simulink library "ExperimentLibrary"  (R2014b)
settings: Solver=ode45  StartTime=0.0  StopTime=10.0  RelTol=1e-3
libraries: simulink x16, ExperimentLibrary x10, simulink_extras x2
settings Model: CovModelRefEnable=off  CovSFcnEnable=on  Creator=oortg  LastModifiedBy=OortG

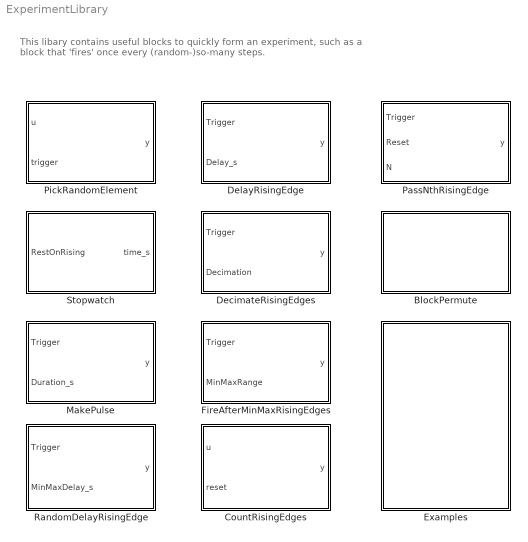
== system ExperimentLibrary ==
  note: This libary contains useful blocks to quickly form an experiment, such as a block that 'fires' once every (random-)so-many steps.
  BlockPermute : Subsystem
  CountRisingEdges : MATLAB Function  TreatAsAtomicUnit=on
      settings: PermitHierarchicalResolution=ParametersOnly
  DecimateRisingEdges : Subsystem
  DelayRisingEdge : Subsystem
  Examples : Subsystem
  FireAfterMinMaxRisingEdges : Subsystem
  MakePulse : Subsystem
  PassNthRisingEdge : Subsystem
  PickRandomElement : MATLAB Function  TreatAsAtomicUnit=on
      settings: PermitHierarchicalResolution=ParametersOnly
  RandomDelayRisingEdge : Subsystem
  Stopwatch : Subsystem

== system ExperimentLibrary/BlockPermute ==
  note: Given vectors in1, in2, in3 and in4, this block will, sequentially, output
      | all combinations of various elements of the inputs in a random order,
      | such that, after N=len(in1)*len(in2)*len(in3)*len(in4)*Ntimes, each combination was
      | output exactly Ntimes times. It is allowed to keep any inX unconnected;
      | this makes the block work for only the remaining inputs.
      |
      | Ntimes should low enough that the total number of combinations offered, N, is
      | less or equal to 1000. If not, Ntimes is reduced until the condition is
      | satisfied. Ntimes can be changed at any time; if so, a new experiment
      | with fresh a random order is started.
      |
      | Each time a rising edge on trigger is encountered, a new combination is
      | generated. Each time a rising edge on trigger_back is generated, the
      | previous combination is output (a simultaneous rising edge on both will
      | continue offering the current combination). For the first time sample of
      | the model (i.e., directly after pressing 'run'), the value of
      | trigger/trigger_back are considered; if nonzero this is seen as a rising
      | edge (this allows for generating the first combination at sample 1
      | already, thus skipping the 'initial value').
      |
      | When N combination are output (i.e., we're finished), a new round is
      | started with a freshly randomized order. The number of completed
      | rounds is returned as 3rd argument in the 'info' output.
      |
      | The first combination is only shown as soon as the first trigger appeared.
      | Because the block needs to output always, there is an initialValue input,
      | which is used as the output values before the first trigger (and also
      | after a enough trigger_back events). It defaults to zero if left empty.
      |
      | It is allowed to change the input values inX during the experiment (though,
      | not the length of the vectors). Internally, only the indices of all combinations
      | are permuted, not the input values themselves. So the block keeps
      | working, keeping in mind which elements of the input arrays had been used
      | or not).
      |
      | On a rising edge of reset, the internal state of the block is reset. It
      | is NOT a level reset though (contrary to most other blocks in the
      | ExperimentLibrary), so even when the reset input is non-zero, the block
      | functions as normal. This allows for applying a rising edge on reset and
      | a rising edge on trigger simultaneously, causing the block to initiate a
      | new experiment and start at the first combination right away (skipping
      | the initial value). Identically, changing Ntimes simultaneously to a rising
      | edge of trigger initiates a new experiment and starts at the first
      | combination too.
      |
      | The info output has the following elements, which are useful for checking
      | how far you are in the experiment:
      |   - number of combinations done in current round
      |   - maximum number of combination (N in the above description)
      |   - Number of full rounds done (if more than N combination were output,
      |     this is nonzero. You can use this to stop your experiment after all
      |     combination have been done Ntimes times, for example).
  BlockPermute_1_Input : Subsystem
  BlockPermute_2_Inputs : Subsystem
  BlockPermute_3_Inputs : Subsystem
  BlockPermute_4_Inputs : Subsystem

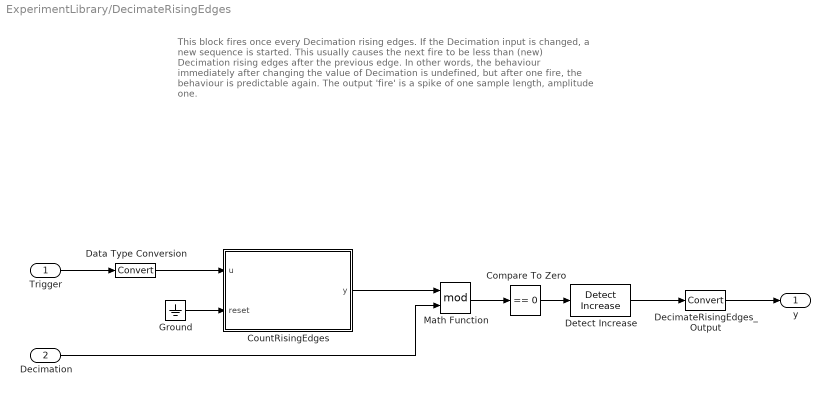
== system ExperimentLibrary/DecimateRisingEdges ==
  note: This block fires once every Decimation rising edges.
      |
      | If the Decimation input is changed, a new sequence
      | is started. This usually causes the next fire to be less than (new) Decimation
      | rising edges after the previous edge. In other words, the behaviour immediately
      | after changing the value of Decimation is undefined, but after one fire, the
      | behaviour is predictable again.
      |
      | The output 'fire' is a spike of one sample length, amplitude one.
  Trigger : Inport
  Decimation : Inport  Port=2
  Compare To Zero : simulink/Logic and Bit Operations/Compare To Zero  relop===  OutDataTypeStr=boolean
  CountRisingEdges : MATLAB Function  TreatAsAtomicUnit=on
      settings: PermitHierarchicalResolution=ParametersOnly
  Data Type Conversion : DataTypeConversion
  DecimateRisingEdges_Output : DataTypeConversion
  Detect Increase : simulink/Logic and Bit Operations/Detect Increase  vinit=1  InputProcessing=Inherited  OutDataTypeStr=boolean
  Ground : Ground
  Math Function : Math  Operator=mod  SaturateOnIntegerOverflow=on
  y : Outport
  wires:
  Compare To Zero/1 -> Detect Increase/1
  Detect Increase/1 -> DecimateRisingEdges_Output/1
  Math Function/1 -> Compare To Zero/1
  Ground/1 -> CountRisingEdges/2(reset)
  CountRisingEdges/1(y) -> Math Function/1
  Trigger/1 -> Data Type Conversion/1
  DecimateRisingEdges_Output/1 -> y/1
  Data Type Conversion/1 -> CountRisingEdges/1(u)
  Decimation/1 -> Math Function/2

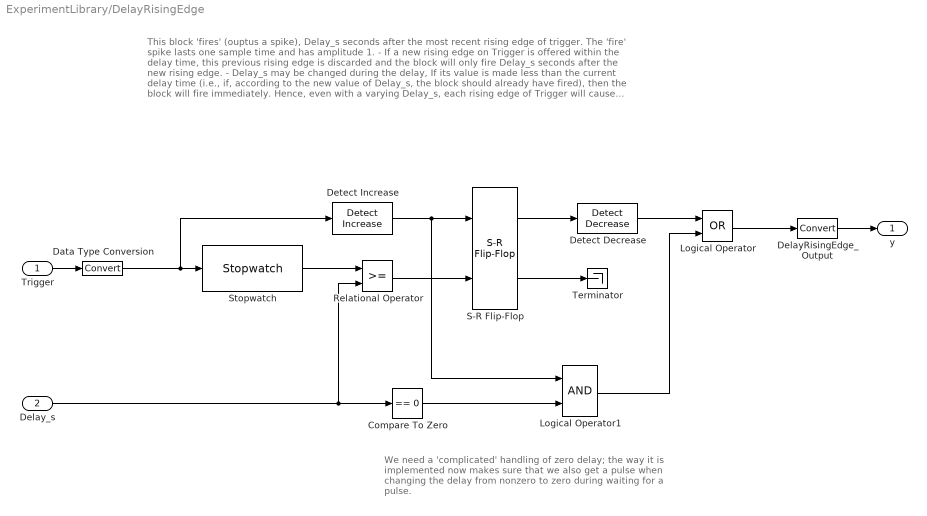
== system ExperimentLibrary/DelayRisingEdge ==
  note: This block 'fires' (ouptus a spike), Delay_s seconds after the most recent rising edge of trigger.
      |
      | The 'fire' spike lasts one sample time and has amplitude 1.
      | - If a new rising edge on Trigger is offered within the delay time, this previous rising edge is
      | discarded and the block will only fire Delay_s seconds after the new rising edge.
      | - Delay_s may be changed during the delay, If its value is made less than the current delay time (i.e.,
      | if, according to the new value of Delay_s, the block should already have fired), then the block will fire
      | immediately. Hence, even with a varying Delay_s, each rising edge of Trigger will cause exactly one fire on the
      | output (unless a new rising edge is offered before the delay time ended).
      | - A delay of zero seconds is handled correctly.
  note: We need a 'complicated' handling of zero delay; the way it is implemented
      | now makes sure that we also get a pulse when changing the delay from nonzero
      | to zero during waiting for a pulse.
  Trigger : Inport
  Delay_s : Inport  Port=2
  Compare To Zero : simulink/Logic and Bit Operations/Compare To Zero  relop===  OutDataTypeStr=boolean
  Data Type Conversion : DataTypeConversion
  DelayRisingEdge_Output : DataTypeConversion
  Detect Decrease : simulink/Logic and Bit Operations/Detect Decrease  vinit=0.0  InputProcessing=Inherited  OutDataTypeStr=boolean
  Detect Increase : simulink/Logic and Bit Operations/Detect Increase  vinit=0.0  InputProcessing=Inherited  OutDataTypeStr=boolean
  Logical Operator : Logic  Operator=OR  AllPortsSameDT=off  OutDataTypeStr=boolean
  Logical Operator1 : Logic  AllPortsSameDT=off  OutDataTypeStr=boolean
  Relational Operator : RelationalOperator  OutDataTypeStr=boolean
  S-R Flip-Flop : simulink_extras/Flip Flops/S-R Flip-Flop  initial_condition=0
  Stopwatch : ExperimentLibrary/Stopwatch
  Terminator : Terminator
  y : Outport
  wires:
  Logical Operator1/1 -> Logical Operator/2
  Detect Decrease/1 -> Logical Operator/1
  Compare To Zero/1 -> Logical Operator1/2
  Logical Operator/1 -> DelayRisingEdge_Output/1
  S-R Flip-Flop/1 -> Detect Decrease/1
  Detect Increase/1 -> S-R Flip-Flop/1, Logical Operator1/1
  Relational Operator/1 -> S-R Flip-Flop/2
  Trigger/1 -> Data Type Conversion/1
  Stopwatch/1 -> Relational Operator/1
  S-R Flip-Flop/2 -> Terminator/1
  DelayRisingEdge_Output/1 -> y/1
  Data Type Conversion/1 -> Detect Increase/1, Stopwatch/1
  Delay_s/1 -> Compare To Zero/1, Relational Operator/2

== system ExperimentLibrary/Examples ==
  Example1 : Subsystem

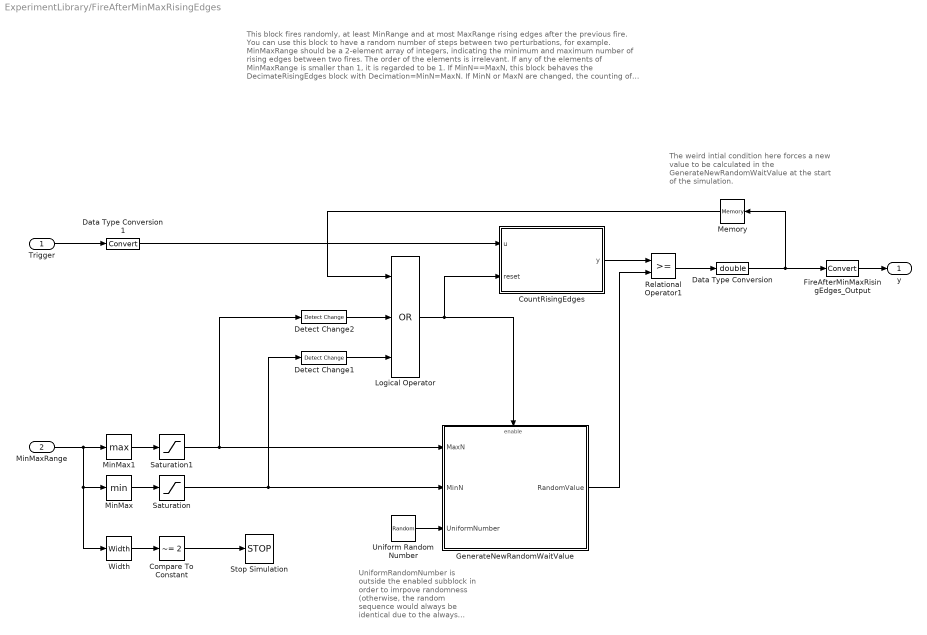
== system ExperimentLibrary/FireAfterMinMaxRisingEdges ==
  note: This block fires randomly, at least MinRange and at most MaxRange rising edges after the previous fire.
      |
      | You can use this block to have a random number of steps between two perturbations, for example.
      |
      | MinMaxRange should be a 2-element array of integers, indicating the minimum and maximum number
      | of rising edges between two fires. The order of the elements is irrelevant.
      |
      | If any of the elements of MinMaxRange is smaller than 1, it is regarded to be 1.
      | If MinN==MaxN, this block behaves the DecimateRisingEdges block with Decimation=MinN=MaxN.
      | If MinN or MaxN are changed, the counting of rising edges is reset (i.e., after a change of MinN or MaxN,
      | it takes MinN to MaxN rising edges before the block fires).
      |
      | The output 'fire' is a spike of one sample length, amplitude one.
  note: UniformRandomNumber is outside the enabled subblock in order to imrpove randomness (otherwise, the random sequence would always be identical due to the always identical seed).
  note: The weird intial condition here forces a new value to be calculated in the GenerateNewRandomWaitValue at the start of the simulation.
  Trigger : Inport
  MinMaxRange : Inport  Port=2
  Compare To Constant : simulink/Logic and Bit Operations/Compare To Constant  relop=~=  const=2  OutDataTypeStr=boolean
  CountRisingEdges : MATLAB Function  TreatAsAtomicUnit=on
      settings: PermitHierarchicalResolution=ParametersOnly
  Data Type Conversion : DataTypeConversion  OutDataTypeStr=double
  Data Type Conversion1 : DataTypeConversion
  Detect Change1 : simulink/Logic and Bit Operations/Detect Change  vinit=0  InputProcessing=Inherited  OutDataTypeStr=boolean
  Detect Change2 : simulink/Logic and Bit Operations/Detect Change  vinit=0  InputProcessing=Inherited  OutDataTypeStr=boolean
  FireAfterMinMaxRisingEdges_Output : DataTypeConversion
  GenerateNewRandomWaitValue : Subsystem
  Logical Operator : Logic  Operator=OR  Inputs=3  AllPortsSameDT=off  OutDataTypeStr=boolean
  Memory : Memory  X0=-32893
  MinMax : MinMax
  MinMax1 : MinMax  Function=max
  Relational Operator1 : RelationalOperator  OutDataTypeStr=boolean
  Saturation : Saturate  UpperLimit=inf  LowerLimit=1
  Saturation1 : Saturate  UpperLimit=inf  LowerLimit=1
  Stop Simulation : Stop
  Uniform Random Number : UniformRandomNumber  Minimum=0
  Width : Width
  y : Outport
  wires:
  Uniform Random Number/1 -> GenerateNewRandomWaitValue/3(UniformNumber)
  Compare To Constant/1 -> Stop Simulation/1
  Width/1 -> Compare To Constant/1
  Saturation1/1 -> GenerateNewRandomWaitValue/1(MaxN), Detect Change2/1
  Saturation/1 -> GenerateNewRandomWaitValue/2(MinN), Detect Change1/1
  MinMax1/1 -> Saturation1/1
  Data Type Conversion/1 -> Memory/1, FireAfterMinMaxRisingEdges_Output/1
  Logical Operator/1 -> CountRisingEdges/2(reset), GenerateNewRandomWaitValue/Enable
  Memory/1 -> Logical Operator/1
  Detect Change1/1 -> Logical Operator/3
  Detect Change2/1 -> Logical Operator/2
  CountRisingEdges/1(y) -> Relational Operator1/1
  GenerateNewRandomWaitValue/1(RandomValue) -> Relational Operator1/2
  MinMaxRange/1 -> MinMax1/1, MinMax/1, Width/1
  MinMax/1 -> Saturation/1
  Relational Operator1/1 -> Data Type Conversion/1
  Trigger/1 -> Data Type Conversion1/1
  FireAfterMinMaxRisingEdges_Output/1 -> y/1
  Data Type Conversion1/1 -> CountRisingEdges/1(u)

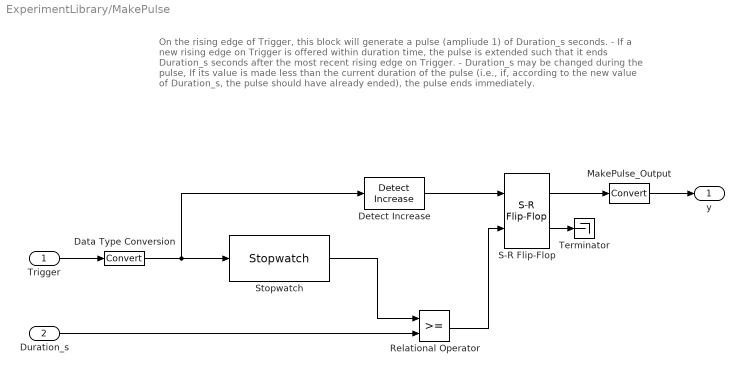
== system ExperimentLibrary/MakePulse ==
  note: On the rising edge of Trigger, this block will generate a pulse (ampliude 1) of Duration_s seconds.
      |
      | - If a new rising edge on Trigger is offered within duration time, the pulse is extended such that it
      |   ends Duration_s seconds after the most recent rising edge on Trigger.
      | - Duration_s may be changed during the pulse, If its value is made less than the current duration of the pulse
      | (i.e., if, according to the new value of Duration_s, the pulse should have already ended), the pulse ends immediately.
  Trigger : Inport
  Duration_s : Inport  Port=2
  Data Type Conversion : DataTypeConversion
  Detect Increase : simulink/Logic and Bit Operations/Detect Increase  vinit=0.0  InputProcessing=Inherited  OutDataTypeStr=boolean
  MakePulse_Output : DataTypeConversion
  Relational Operator : RelationalOperator  OutDataTypeStr=boolean
  S-R Flip-Flop : simulink_extras/Flip Flops/S-R Flip-Flop  initial_condition=0
  Stopwatch : ExperimentLibrary/Stopwatch
  Terminator : Terminator
  y : Outport
  wires:
  S-R Flip-Flop/1 -> MakePulse_Output/1
  Detect Increase/1 -> S-R Flip-Flop/1
  Relational Operator/1 -> S-R Flip-Flop/2
  Trigger/1 -> Data Type Conversion/1
  Stopwatch/1 -> Relational Operator/1
  S-R Flip-Flop/2 -> Terminator/1
  MakePulse_Output/1 -> y/1
  Data Type Conversion/1 -> Stopwatch/1, Detect Increase/1
  Duration_s/1 -> Relational Operator/2

== system ExperimentLibrary/PassNthRisingEdge ==
  note: This block passes the N'th rising edge of Trigger (after doing this, the internal counter
      | is NOT reset, so if no external reset signal is given, only one rising edge is passed).
      |
      | When Reset is high (level-reset), the counting is reset; after Reset going low again,
      | the counting starts from 0.
      |
      | If N is changed during the counting, the block acts as  if N had always been on the new
      | value (i.e., if N was 2, and after 3 rising edges N is made 5, the block already had fired at 2
      | and will fire again at 5 rising edges).
  Trigger : Inport
  Reset : Inport  Port=2
  N : Inport  Port=3
  CountRisingEdges : MATLAB Function  TreatAsAtomicUnit=on
      settings: PermitHierarchicalResolution=ParametersOnly
  Data Type Conversion : DataTypeConversion
  Data Type Conversion1 : DataTypeConversion
  Detect Increase : simulink/Logic and Bit Operations/Detect Increase  vinit=0.0  InputProcessing=Inherited  OutDataTypeStr=boolean
  PassNthRisingEdge_Output : DataTypeConversion
  Relational Operator : RelationalOperator  Operator===  OutDataTypeStr=boolean
  y : Outport
  wires:
  Relational Operator/1 -> Detect Increase/1
  N/1 -> Relational Operator/2
  CountRisingEdges/1(y) -> Relational Operator/1
  Detect Increase/1 -> PassNthRisingEdge_Output/1
  Reset/1 -> Data Type Conversion1/1
  Trigger/1 -> Data Type Conversion/1
  PassNthRisingEdge_Output/1 -> y/1
  Data Type Conversion/1 -> CountRisingEdges/1(u)
  Data Type Conversion1/1 -> CountRisingEdges/2(reset)

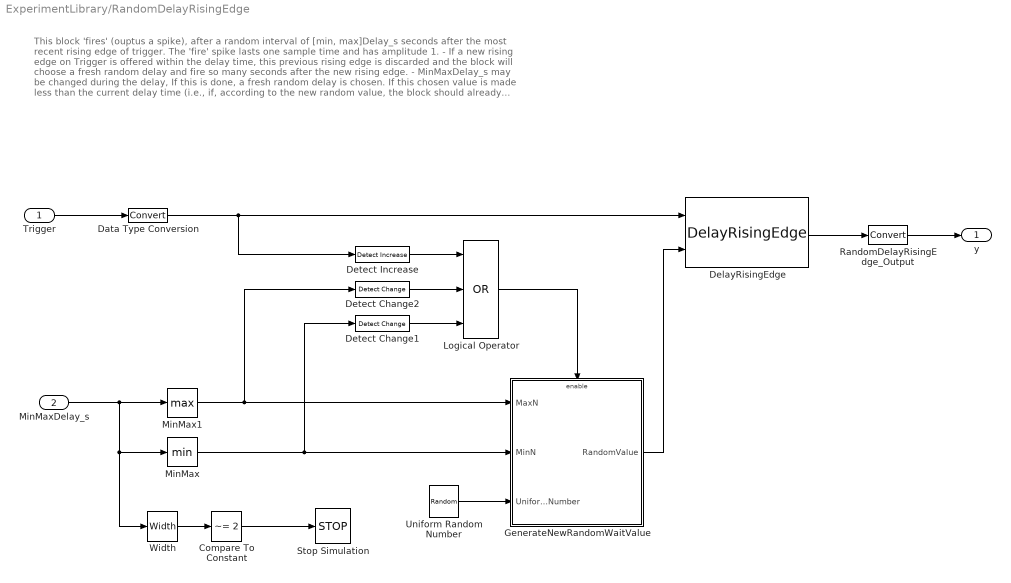
== system ExperimentLibrary/RandomDelayRisingEdge ==
  note: This block 'fires' (ouptus a spike), after a random interval of [min, max]Delay_s seconds after the most recent rising edge of trigger.
      |
      | The 'fire' spike lasts one sample time and has amplitude 1.
      | - If a new rising edge on Trigger is offered within the delay time, this previous rising edge is discarded and the block will choose a fresh random delay and fire so many seconds after the new rising edge.
      | - MinMaxDelay_s may be changed during the delay, If this is done, a fresh random delay is chosen. If this chosen value is made less than the current delay time (i.e., if, according to the new random value, the block should already have fired), then the block will fire immediately. Hence, even with when varying the MinMaxDelay_s input, each rising edge of Trigger will cause exactly one fire on the output (unless a new rising edge is offered before the delay time ended).
      | - A minimum delay of 0 seconds is allowed.
  Trigger : Inport
  MinMaxDelay_s : Inport  Port=2
  Compare To Constant : simulink/Logic and Bit Operations/Compare To Constant  relop=~=  const=2  OutDataTypeStr=boolean
  Data Type Conversion : DataTypeConversion
  DelayRisingEdge : ExperimentLibrary/DelayRisingEdge
  Detect Change1 : simulink/Logic and Bit Operations/Detect Change  vinit=0  InputProcessing=Inherited  OutDataTypeStr=boolean
  Detect Change2 : simulink/Logic and Bit Operations/Detect Change  vinit=0  InputProcessing=Inherited  OutDataTypeStr=boolean
  Detect Increase : simulink/Logic and Bit Operations/Detect Increase  vinit=0.0  InputProcessing=Inherited  OutDataTypeStr=boolean
  GenerateNewRandomWaitValue : Subsystem
  Logical Operator : Logic  Operator=OR  Inputs=3  AllPortsSameDT=off  OutDataTypeStr=boolean
  MinMax : MinMax
  MinMax1 : MinMax  Function=max
  RandomDelayRisingEdge_Output : DataTypeConversion
  Stop Simulation : Stop
  Uniform Random Number : UniformRandomNumber  Minimum=0
  Width : Width
  y : Outport
  wires:
  Data Type Conversion/1 -> DelayRisingEdge/1, Detect Increase/1
  Trigger/1 -> Data Type Conversion/1
  RandomDelayRisingEdge_Output/1 -> y/1
  Detect Increase/1 -> Logical Operator/1
  GenerateNewRandomWaitValue/1(RandomValue) -> DelayRisingEdge/2
  Logical Operator/1 -> GenerateNewRandomWaitValue/Enable
  MinMaxDelay_s/1 -> Width/1, MinMax/1, MinMax1/1
  Width/1 -> Compare To Constant/1
  Compare To Constant/1 -> Stop Simulation/1
  Detect Change2/1 -> Logical Operator/2
  Detect Change1/1 -> Logical Operator/3
  MinMax/1 -> Detect Change1/1, GenerateNewRandomWaitValue/2(MinN)
  MinMax1/1 -> Detect Change2/1, GenerateNewRandomWaitValue/1(MaxN)
  Uniform Random Number/1 -> GenerateNewRandomWaitValue/3(UniformNumber)
  DelayRisingEdge/1 -> RandomDelayRisingEdge_Output/1

== system ExperimentLibrary/Stopwatch ==
  RestOnRising : Inport
  Clock : Clock
  Data Type Conversion : DataTypeConversion
  SampleAndHold : Subsystem
  Sum : Sum  Inputs=-+|
  time_s : Outport
  wires:
  Sum/1 -> time_s/1
  SampleAndHold/1(Out) -> Sum/1
  RestOnRising/1 -> Data Type Conversion/1
  Clock/1 -> SampleAndHold/1(In), Sum/2
  Data Type Conversion/1 -> SampleAndHold/Trigger

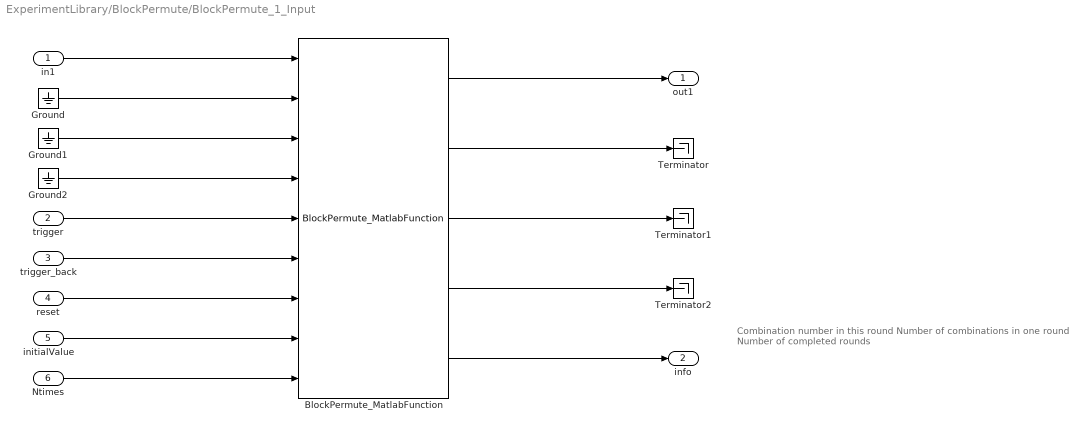
== system ExperimentLibrary/BlockPermute/BlockPermute_1_Input ==
  note: Combination number in this round
      | Number of combinations in one round
      | Number of completed rounds
  in1 : Inport
  trigger : Inport  Port=2
  trigger_back : Inport  Port=3
  reset : Inport  Port=4
  initialValue : Inport  Port=5
  Ntimes : Inport  Port=6
  BlockPermute_MatlabFunction : ExperimentLibrary/BlockPermute/BlockPermute_4_Inputs/BlockPermute_MatlabFunction
  Ground : Ground
  Ground1 : Ground
  Ground2 : Ground
  Terminator : Terminator
  Terminator1 : Terminator
  Terminator2 : Terminator
  out1 : Outport
  info : Outport  Port=2
  wires:
  BlockPermute_MatlabFunction/5 -> info/1
  BlockPermute_MatlabFunction/2 -> Terminator/1
  BlockPermute_MatlabFunction/1 -> out1/1
  Ntimes/1 -> BlockPermute_MatlabFunction/9
  initialValue/1 -> BlockPermute_MatlabFunction/8
  reset/1 -> BlockPermute_MatlabFunction/7
  trigger_back/1 -> BlockPermute_MatlabFunction/6
  trigger/1 -> BlockPermute_MatlabFunction/5
  Ground2/1 -> BlockPermute_MatlabFunction/4
  Ground1/1 -> BlockPermute_MatlabFunction/3
  Ground/1 -> BlockPermute_MatlabFunction/2
  in1/1 -> BlockPermute_MatlabFunction/1
  BlockPermute_MatlabFunction/3 -> Terminator1/1
  BlockPermute_MatlabFunction/4 -> Terminator2/1

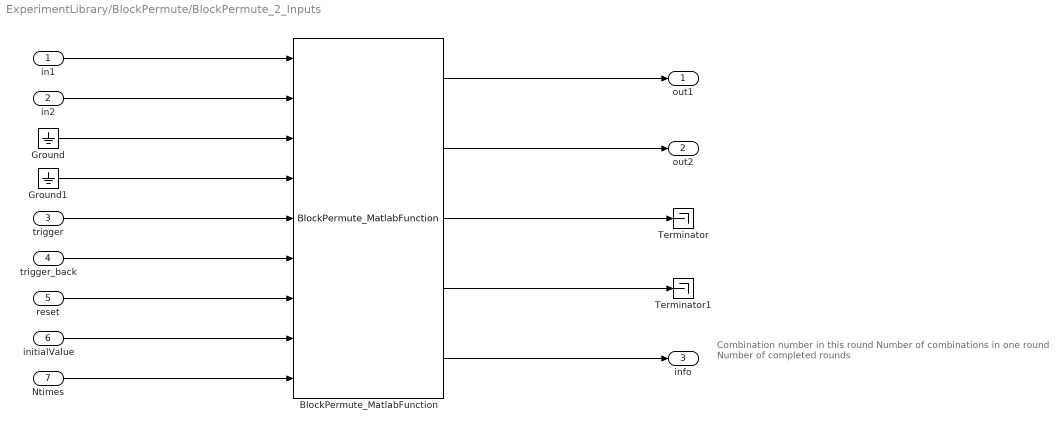
== system ExperimentLibrary/BlockPermute/BlockPermute_2_Inputs ==
  note: Combination number in this round
      | Number of combinations in one round
      | Number of completed rounds
  in1 : Inport
  in2 : Inport  Port=2
  trigger : Inport  Port=3
  trigger_back : Inport  Port=4
  reset : Inport  Port=5
  initialValue : Inport  Port=6
  Ntimes : Inport  Port=7
  BlockPermute_MatlabFunction : ExperimentLibrary/BlockPermute/BlockPermute_4_Inputs/BlockPermute_MatlabFunction
  Ground : Ground
  Ground1 : Ground
  Terminator : Terminator
  Terminator1 : Terminator
  out1 : Outport
  out2 : Outport  Port=2
  info : Outport  Port=3
  wires:
  in1/1 -> BlockPermute_MatlabFunction/1
  in2/1 -> BlockPermute_MatlabFunction/2
  Ground/1 -> BlockPermute_MatlabFunction/3
  Ground1/1 -> BlockPermute_MatlabFunction/4
  trigger/1 -> BlockPermute_MatlabFunction/5
  trigger_back/1 -> BlockPermute_MatlabFunction/6
  reset/1 -> BlockPermute_MatlabFunction/7
  initialValue/1 -> BlockPermute_MatlabFunction/8
  Ntimes/1 -> BlockPermute_MatlabFunction/9
  BlockPermute_MatlabFunction/1 -> out1/1
  BlockPermute_MatlabFunction/2 -> out2/1
  BlockPermute_MatlabFunction/3 -> Terminator/1
  BlockPermute_MatlabFunction/4 -> Terminator1/1
  BlockPermute_MatlabFunction/5 -> info/1

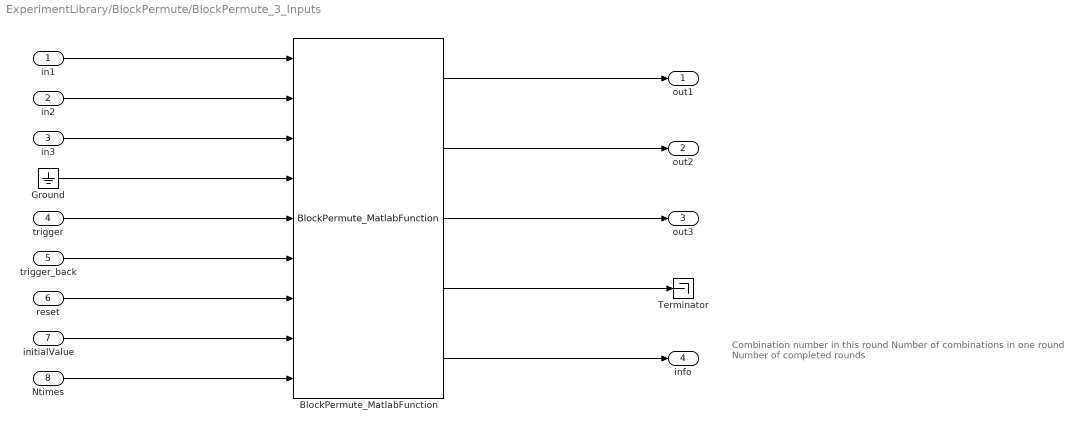
== system ExperimentLibrary/BlockPermute/BlockPermute_3_Inputs ==
  note: Combination number in this round
      | Number of combinations in one round
      | Number of completed rounds
  in1 : Inport
  in2 : Inport  Port=2
  in3 : Inport  Port=3
  trigger : Inport  Port=4
  trigger_back : Inport  Port=5
  reset : Inport  Port=6
  initialValue : Inport  Port=7
  Ntimes : Inport  Port=8
  BlockPermute_MatlabFunction : ExperimentLibrary/BlockPermute/BlockPermute_4_Inputs/BlockPermute_MatlabFunction
  Ground : Ground
  Terminator : Terminator
  out1 : Outport
  out2 : Outport  Port=2
  out3 : Outport  Port=3
  info : Outport  Port=4
  wires:
  BlockPermute_MatlabFunction/5 -> info/1
  BlockPermute_MatlabFunction/4 -> Terminator/1
  BlockPermute_MatlabFunction/3 -> out3/1
  BlockPermute_MatlabFunction/2 -> out2/1
  BlockPermute_MatlabFunction/1 -> out1/1
  Ntimes/1 -> BlockPermute_MatlabFunction/9
  initialValue/1 -> BlockPermute_MatlabFunction/8
  reset/1 -> BlockPermute_MatlabFunction/7
  trigger_back/1 -> BlockPermute_MatlabFunction/6
  trigger/1 -> BlockPermute_MatlabFunction/5
  Ground/1 -> BlockPermute_MatlabFunction/4
  in3/1 -> BlockPermute_MatlabFunction/3
  in2/1 -> BlockPermute_MatlabFunction/2
  in1/1 -> BlockPermute_MatlabFunction/1

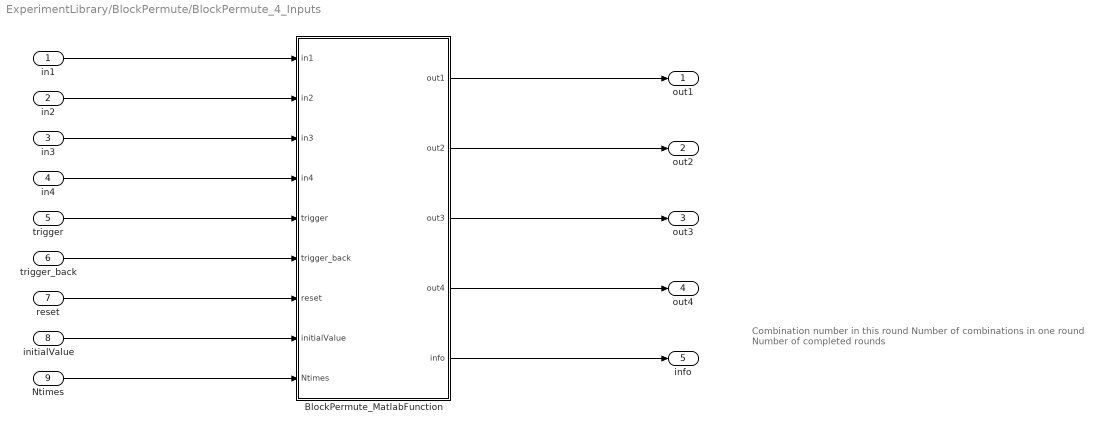
== system ExperimentLibrary/BlockPermute/BlockPermute_4_Inputs ==
  note: Combination number in this round
      | Number of combinations in one round
      | Number of completed rounds
  in1 : Inport
  in2 : Inport  Port=2
  in3 : Inport  Port=3
  in4 : Inport  Port=4
  trigger : Inport  Port=5
  trigger_back : Inport  Port=6
  reset : Inport  Port=7
  initialValue : Inport  Port=8
  Ntimes : Inport  Port=9
  BlockPermute_MatlabFunction : Subsystem
  out1 : Outport
  out2 : Outport  Port=2
  out3 : Outport  Port=3
  out4 : Outport  Port=4
  info : Outport  Port=5
  wires:
  in1/1 -> BlockPermute_MatlabFunction/1(in1)
  in2/1 -> BlockPermute_MatlabFunction/2(in2)
  in3/1 -> BlockPermute_MatlabFunction/3(in3)
  in4/1 -> BlockPermute_MatlabFunction/4(in4)
  trigger/1 -> BlockPermute_MatlabFunction/5(trigger)
  trigger_back/1 -> BlockPermute_MatlabFunction/6(trigger_back)
  reset/1 -> BlockPermute_MatlabFunction/7(reset)
  initialValue/1 -> BlockPermute_MatlabFunction/8(initialValue)
  Ntimes/1 -> BlockPermute_MatlabFunction/9(Ntimes)
  BlockPermute_MatlabFunction/1(out1) -> out1/1
  BlockPermute_MatlabFunction/2(out2) -> out2/1
  BlockPermute_MatlabFunction/3(out3) -> out3/1
  BlockPermute_MatlabFunction/4(out4) -> out4/1
  BlockPermute_MatlabFunction/5(info) -> info/1

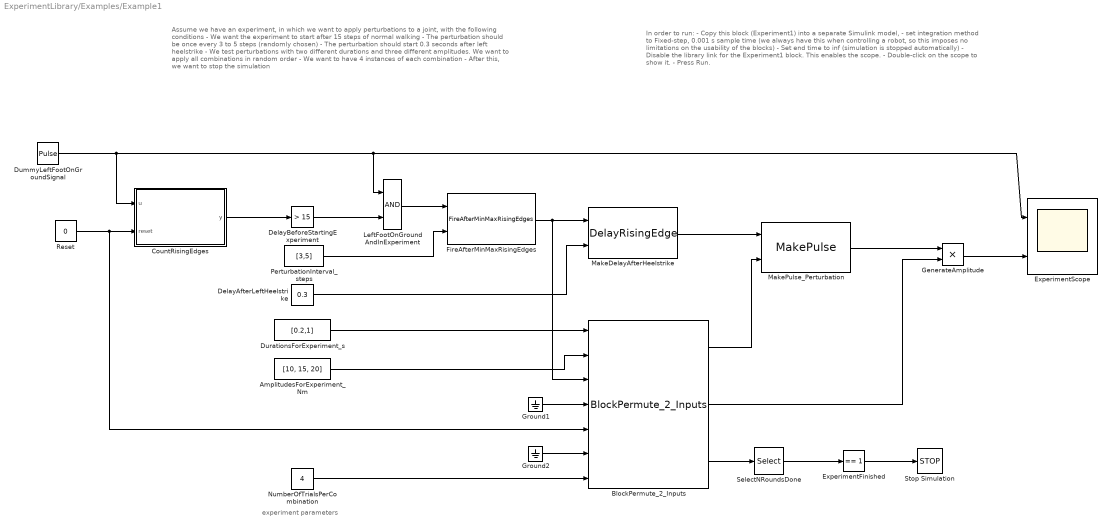
== system ExperimentLibrary/Examples/Example1 ==
  note: In order to run:
      | - Copy this block (Experiment1) into a separate Simulink model,
      | - set integration method to Fixed-step, 0.001 s sample time (we always have this when
      | controlling a robot, so this imposes no limitations on the usability of the blocks)
      | - Set end time to inf (simulation is stopped automatically)
      | - Disable the library link for the Experiment1 block. This enables the scope.
      | - Double-click on the scope to show it.
      | - Press Run.
  note: Assume we have an experiment, in which we want to apply perturbations to a joint, with the following conditions
      | - We want the experiment to start after 15 steps of normal walking
      | - The perturbation should be once every 3 to 5 steps (randomly chosen)
      | - The perturbation should start 0.3 seconds after left heelstrike
      | - We test perturbations with two different durations and three different amplitudes. We want to apply all combinations in random order
      | - We want to have 4 instances of each combination
      | - After this, we want to stop the simulation
  note: experiment
      | parameters
  AmplitudesForExperiment_Nm : Constant  Value=[10, 15, 20]
  BlockPermute_2_Inputs : ExperimentLibrary/BlockPermute/BlockPermute_2_Inputs
  CountRisingEdges : MATLAB Function  TreatAsAtomicUnit=on
      settings: PermitHierarchicalResolution=ParametersOnly
  DelayAfterLeftHeelstrike : Constant  Value=0.3
  DelayBeforeStartingExperiment : simulink/Logic and Bit Operations/Compare To Constant  relop=>  const=15  OutDataTypeStr=boolean
  DummyLeftFootOnGroundSignal : DiscretePulseGenerator  PulseType=Time based  Period=1.8  PulseWidth=60
  DurationsForExperiment_s : Constant  Value=[0.2,1]
  ExperimentFinished : simulink/Logic and Bit Operations/Compare To Constant  relop===  const=1  OutDataTypeStr=boolean
  ExperimentScope : Scope  NumInputPorts=2
      settings: TimeRange=auto  MaxDataPoints=5000  SaveToWorkspace=off  YMin=-0.125~-2.5  YMax=1.125~22.5  SampleTime=-1
  FireAfterMinMaxRisingEdges : ExperimentLibrary/FireAfterMinMaxRisingEdges
  GenerateAmplitude : Product
  Ground1 : Ground
  Ground2 : Ground
  LeftFootOnGround AndInExperiment : Logic  AllPortsSameDT=off  OutDataTypeStr=boolean
  MakeDelayAfterHeelstrike : ExperimentLibrary/DelayRisingEdge
  MakePulse_Perturbation : ExperimentLibrary/MakePulse
  NumberOfTrialsPerCombination : Constant  Value=4
  PerturbationInterval_steps : Constant  Value=[3,5]
  Reset : Constant  Value=0
  SelectNRoundsDone : Selector  InputPortWidth=3  IndexOptions=Index vector (dialog)  Indices=3  OutputSizes=1
  Stop Simulation : Stop
  wires:
  PerturbationInterval_steps/1 -> FireAfterMinMaxRisingEdges/2
  LeftFootOnGround AndInExperiment/1 -> FireAfterMinMaxRisingEdges/1
  BlockPermute_2_Inputs/1 -> MakePulse_Perturbation/2
  DelayAfterLeftHeelstrike/1 -> MakeDelayAfterHeelstrike/2
  SelectNRoundsDone/1 -> ExperimentFinished/1
  BlockPermute_2_Inputs/3 -> SelectNRoundsDone/1
  MakePulse_Perturbation/1 -> GenerateAmplitude/1
  DelayBeforeStartingExperiment/1 -> LeftFootOnGround AndInExperiment/2
  Reset/1 -> CountRisingEdges/2(reset), BlockPermute_2_Inputs/5
  DummyLeftFootOnGroundSignal/1 -> LeftFootOnGround AndInExperiment/1, ExperimentScope/1, CountRisingEdges/1(u)
  CountRisingEdges/1(y) -> DelayBeforeStartingExperiment/1
  ExperimentFinished/1 -> Stop Simulation/1
  DurationsForExperiment_s/1 -> BlockPermute_2_Inputs/1
  BlockPermute_2_Inputs/2 -> GenerateAmplitude/2
  Ground2/1 -> BlockPermute_2_Inputs/6
  NumberOfTrialsPerCombination/1 -> BlockPermute_2_Inputs/7
  GenerateAmplitude/1 -> ExperimentScope/2
  MakeDelayAfterHeelstrike/1 -> MakePulse_Perturbation/1
  AmplitudesForExperiment_Nm/1 -> BlockPermute_2_Inputs/2
  FireAfterMinMaxRisingEdges/1 -> MakeDelayAfterHeelstrike/1, BlockPermute_2_Inputs/3
  Ground1/1 -> BlockPermute_2_Inputs/4

== system ExperimentLibrary/FireAfterMinMaxRisingEdges/GenerateNewRandomWaitValue ==
  note: MinN<=thisValue<=MaxValue,
      | uniformly distributed
  MaxN : Inport
  MinN : Inport  Port=2
  UniformNumber : Inport  Port=3
  Enable : EnablePort
  Add : Sum  Inputs=+-+
  Add1 : Sum
  One : Constant
  Product : Product
  Rounding Function : Rounding
  RandomValue : Outport
  wires:
  MinN/1 -> Add/2, Add1/1
  MaxN/1 -> Add/1
  One/1 -> Add/3
  Product/1 -> Rounding Function/1
  Rounding Function/1 -> Add1/2
  UniformNumber/1 -> Product/2
  Add1/1 -> RandomValue/1
  Add/1 -> Product/1

== system ExperimentLibrary/RandomDelayRisingEdge/GenerateNewRandomWaitValue ==
  note: MinN<=thisValue<=MaxValue,
      | uniformly distributed
  MaxN : Inport
  MinN : Inport  Port=2
  UniformNumber : Inport  Port=3
  Enable : EnablePort
  Add : Sum  Inputs=+-
  Add1 : Sum
  Product : Product
  RandomValue : Outport
  wires:
  MinN/1 -> Add/2, Add1/1
  MaxN/1 -> Add/1
  Product/1 -> Add1/2
  UniformNumber/1 -> Product/2
  Add1/1 -> RandomValue/1
  Add/1 -> Product/1

== system ExperimentLibrary/Stopwatch/SampleAndHold ==
  note: Initial output is -100 such that the perturbation generator starts with a zero output
  In : Inport
  Trigger : TriggerPort  PortDimensions=1
  Out : Outport  InitialOutput=[-100]
  wires:
  In/1 -> Out/1

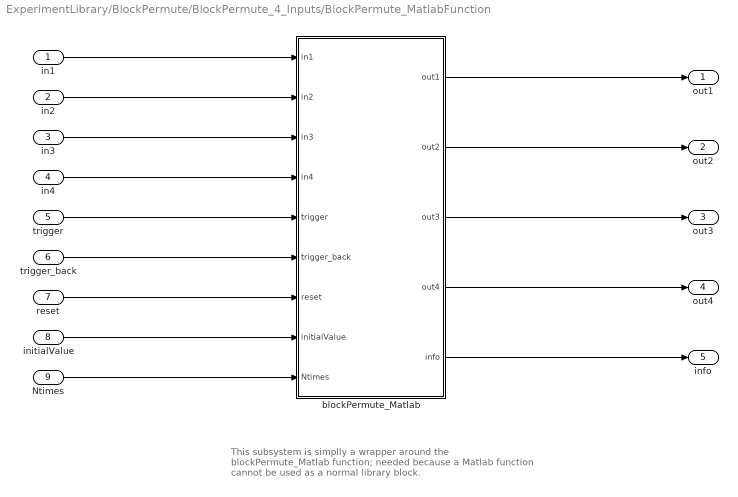
== system ExperimentLibrary/BlockPermute/BlockPermute_4_Inputs/BlockPermute_MatlabFunction ==
  note: This subsystem is simplly a wrapper around the blockPermute_Matlab function; needed because a Matlab function cannot be used as a normal library block.
  in1 : Inport
  in2 : Inport  Port=2
  in3 : Inport  Port=3
  in4 : Inport  Port=4
  trigger : Inport  Port=5
  trigger_back : Inport  Port=6
  reset : Inport  Port=7
  initialValue : Inport  Port=8
  Ntimes : Inport  Port=9
  blockPermute_Matlab : MATLAB Function  TreatAsAtomicUnit=on
      settings: PermitHierarchicalResolution=ParametersOnly
  out1 : Outport
  out2 : Outport  Port=2
  out3 : Outport  Port=3
  out4 : Outport  Port=4
  info : Outport  Port=5
  wires:
  blockPermute_Matlab/2(out2) -> out2/1
  blockPermute_Matlab/1(out1) -> out1/1
  blockPermute_Matlab/4(out4) -> out4/1
  blockPermute_Matlab/5(info) -> info/1
  blockPermute_Matlab/3(out3) -> out3/1
  in2/1 -> blockPermute_Matlab/2(in2)
  trigger_back/1 -> blockPermute_Matlab/6(trigger_back)
  in4/1 -> blockPermute_Matlab/4(in4)
  in3/1 -> blockPermute_Matlab/3(in3)
  Ntimes/1 -> blockPermute_Matlab/9(Ntimes)
  in1/1 -> blockPermute_Matlab/1(in1)
  trigger/1 -> blockPermute_Matlab/5(trigger)
  reset/1 -> blockPermute_Matlab/7(reset)
  initialValue/1 -> blockPermute_Matlab/8(initialValue)

== matlab function ExperimentLibrary/DecimateRisingEdges/CountRisingEdges ==
  data: u input; y output; reset input
function y = CountRisingEdges(u,reset)
%
% Counts the number samples that the signal of u is rising. For
% boolean-like signals, this is identical to counting the number of times
% u goes from low to high. The reset function works as level reset (as long
% as it is high, the output is kept zero).

%#codegen

persistent u_prev_
persistent count_

if isempty(u_prev_)
    u_prev_=u; % Ensures no trigger at start of model
    count_=0;
end;

if reset
    count_ = 0;
else
    if u>u_prev_
        count_=count_+1;
    end;
end;

u_prev_ = u;
y = count_;

== matlab function ExperimentLibrary/FireAfterMinMaxRisingEdges/CountRisingEdges ==
  data: u input; y output; reset input
function y = CountRisingEdges(u,reset)
%
% Counts the number samples that the signal of u is rising. For
% boolean-like signals, this is identical to counting the number of times
% u goes from low to high. The reset function works as level reset (as long
% as it is high, the output is kept zero).

%#codegen

persistent u_prev_
persistent count_

if isempty(u_prev_)
    u_prev_=u; % Ensures no trigger at start of model
    count_=0;
end;

if reset
    count_ = 0;
else
    if u>u_prev_
        count_=count_+1;
    end;
end;

u_prev_ = u;
y = count_;

== matlab function ExperimentLibrary/PassNthRisingEdge/CountRisingEdges ==
  data: u input; y output; reset input
function y = CountRisingEdges(u,reset)
%
% Counts the number samples that the signal of u is rising. For
% boolean-like signals, this is identical to counting the number of times
% u goes from low to high. The reset function works as level reset (as long
% as it is high, the output is kept zero).

%#codegen

persistent u_prev_
persistent count_

if isempty(u_prev_)
    u_prev_=u; % Ensures no trigger at start of model
    count_=0;
end;

if reset
    count_ = 0;
else
    if u>u_prev_
        count_=count_+1;
    end;
end;

u_prev_ = u;
y = count_;

== matlab function ExperimentLibrary/BlockPermute/BlockPermute_4_Inputs/BlockPermute_MatlabFunction/blockPermute_Matlab ==
  data: in1 input; out1 output; in2 input; in3 input; in4 input; trigger input; trigger_back input; reset input; out2 output; out3 output; out4 output; info output; initialValue input; Ntimes input
function [out1,out2,out3,out4,info]= blockPermute(in1,in2,in3,in4,trigger,trigger_back,reset, initialValue, Ntimes)
%#codegen

% Given vectors in1, in2, in3 and in4, this block will, sequentially, output
% all combinations of various elements of the inputs in a random order,
% such that, after N=len(in1)*len(in2)*len(in3)*len(in4)*Ntimes, each combination was
% output exactly Ntimes times. It is allowed to keep any inX unconnected;
% this makes the block work for only the remaining inputs.
%
% Ntimes should low enough that the total number of combinations offered, N, is
% less or equal to 1000. If not, Ntimes is reduced until the condition is
% satisfied. Ntimes can be changed at any time; if so, a new experiment
% with fresh a random order is started.
%
% Each time a rising edge on trigger is encountered, a new combination is
% generated. Each time a rising edge on trigger_back is generated, the
% previous combination is output (a simultaneous rising edge on both will
% continue offering the current combination). For the first time sample of
% the model (i.e., directly after pressing 'run'), the value of
% trigger/trigger_back are considered; if nonzero this is seen as a rising
% edge (this allows for generating the first combination at sample 1
% already, thus skipping the 'initial value').
%
% When N combination are output (i.e., we're finished), a new round is
% started with a freshly randomized order. The number of completed
% rounds is returned as 3rd argument in the 'info' output.
%
% The first combination is only shown as soon as the first trigger appeared. 
% Because the block needs to output always, there is an initialValue input,
% which is used as the output values before the first trigger (and also
% after a enough trigger_back events). It defaults to zero if left empty.
%
% It is allowed to change the input values inX during the experiment (though,
% not the length of the vectors). Internally, only the indices of all combinations
% are permuted, not the input values themselves. So the block keeps
% working, keeping in mind which elements of the input arrays had been used
% or not).
%
% On a rising edge of reset, the internal state of the block is reset. It
% is NOT a level reset though (contrary to most other blocks in the
% ExperimentLibrary), so even when the reset input is non-zero, the block
% functions as normal. This allows for applying a rising edge on reset and
% a rising edge on trigger simultaneously, causing the block to initiate a
% new experiment and start at the first combination right away (skipping
% the initial value). Identically, changing Ntimes simultaneously to a rising
% edge of trigger initiates a new experiment and starts at the first
% combination too.
%
% The info output has the following elements, which are useful for checking
% how far you are in the experiment:
%   - number of combinations done in current round
%   - maximum number of combination (N in the above description)
%   - Number of full rounds done (if more than N combination were output,
%     this is nonzero. You can use this to stop your experiment after all
%     combination have been done Ntimes times, for example).
%
% 
persistent permutationArray
persistent N % Number of combinations needed
persistent n % Current combination number (or 0 if not yet started)
persistent N1 N2 N3 N4 % Length of inputs in1, in2,in3 and in4
persistent N1234 % Product of N1 .. N4
persistent NRoundsDone
persistent trigger_prev trigger_back_prev reset_prev
persistent Ntimes_prev

% Convert type for compatibility)
trigger = double(trigger);
trigger_back = double(trigger_back);
reset = double(reset);

% By using the random number generator each sample, (as below), we ensure
% that randperm will give different results each time we restart the model
% (since we usually won't reshuffle at exactly the same sample time).
dummy = rand(1);  %#ok<NASGU>

needNewPermutation = 0;

if isempty(permutationArray)
    % Initialize all persistent variables
    permutationArray=zeros(1,1000);
    permutationArray(1) = -1; % Indication that the permutation array wasn't initialized yet
    trigger_prev = 0;
    trigger_back_prev = 0;
    reset_prev = reset;
    Ntimes_prev = Ntimes;
    N1 = length(in1); % Note: an unconnected input defaults to the scalar 0, which has length 1
    N2 = length(in2);
    N3 = length(in3);
    N4 = length(in4);
    N1234 = N1 * N2  * N3 * N4;
    N = N1234 * Ntimes;
    n=0;
    NRoundsDone = 0;
    needNewPermutation = 0; % We'll do the shuffling for the
        % first time when the first trigger occurs. This way, because the
        % first trigger will always be at a different time sample, we
        % ensure pure randomness (not the same 'random' sequence each time
        % we start the model).
end

if Ntimes ~= Ntimes_prev || reset > reset_prev
    % This works, even when reset is high-level. If this is changed at the
    % exact same time instant as trigger, we need to immediately go to the
    % first element, so the order of this and 'if trigger' is important...
    % (same for 
    needNewPermutation = 1;
    n = 0;
    NRoundsDone = 0;
    N = N1234 * Ntimes;
end;

if trigger>trigger_prev
    n = n + 1;
    if permutationArray(1) == -1, needNewPermutation = 1; end; % For initialization for the very first time
end;
if trigger_back>trigger_back_prev
    n = max(0,n - 1);
end;
if n>N
    needNewPermutation = 1;
    n = 1;
    NRoundsDone = NRoundsDone + 1;
end;

if needNewPermutation
    % Then we need to reinitialize the permutation array
    NTimesActual = min(Ntimes, fix(1000/(N1234))); % Makes sure the total number of combinations will not exceed 1000
    % No check whether NTimesActual is nonzero...
    
    N = NTimesActual * N1234;
    permutationArray(1:N) = mod(randperm(N), N1234); % Now it contains the values 0...(N1234-1) NTimesActual times.
end;

if n==0
    l=length(initialValue);
    if l>=1, out1 = initialValue(1); else out1 = 0; end;
    if l>=2, out2 = initialValue(2); else out2 = 0; end;
    if l>=3, out3 = initialValue(3); else out3 = 0; end;
    if l>=4, out4 = initialValue(4); else out4 = 0; end;
else
    % n==1...N
    % now, permutationArray(n) can be used for indexing. It is
    % zero-indexed, and works as follows. Given N1==2, N2==2, N3==2 and
    % N4==1 (thus, 8 permutations), we have (all zero-indexed):
    % index   in1-index   in2-index   in3-index   in4-index
    %  0         0           0           0           0
    %  1         1           0           0           0
    %  2         0           1           0           0
    %  3         1           1           0           0
    %  4         0           0           1           0
    %   .....
    nn = permutationArray(n);
    i1 = mod(nn,N1) + 1; % This is now one-indexed
    i2 = mod( fix(nn/N1), N2) + 1;
    i3 = mod( fix(nn/(N1*N2)), N3) + 1;
    i4 = mod(fix(nn/(N1*N2*N3)),N4) + 1;
    
    out1 = in1(i1);
    out2 = in2(i2);
    out3 = in3(i3);
    out4 = in4(i4);
end;

info = [n;N;NRoundsDone];

trigger_prev = trigger;
trigger_back_prev = trigger_back;
reset_prev = reset;
Ntimes_prev = Ntimes;

== matlab function ExperimentLibrary/Examples/Example1/CountRisingEdges ==
  data: u input; y output; reset input
function y = CountRisingEdges(u,reset)
%
% Counts the number samples that the signal of u is rising. For
% boolean-like signals, this is identical to counting the number of times
% u goes from low to high. The reset function works as level reset (as long
% as it is high, the output is kept zero).

%#codegen

persistent u_prev_
persistent count_

if isempty(u_prev_)
    u_prev_=u; % Ensures no trigger at start of model
    count_=0;
end;

if reset
    count_ = 0;
else
    if u>u_prev_
        count_=count_+1;
    end;
end;

u_prev_ = u;
y = count_;

== matlab function ExperimentLibrary/CountRisingEdges ==
  data: u input; y output; reset input
function y = CountRisingEdges(u,reset)
%
% Counts the number samples that the signal of u is rising. For
% boolean-like signals, this is identical to counting the number of times
% u goes from low to high. The reset function works as level reset (as long
% as it is high, the output is kept zero).

%#codegen

persistent u_prev_
persistent count_

if isempty(u_prev_)
    u_prev_=u; % Ensures no trigger at start of model
    count_=0;
end;

if reset
    count_ = 0;
else
    if u>u_prev_
        count_=count_+1;
    end;
end;

u_prev_ = u;
y = count_;

== matlab function ExperimentLibrary/PickRandomElement ==
  data: u input; y output; trigger input
function y = fcn(u, trigger)
%
% Outputs a random element of the u input (which should be a vector).
% On rising edge of trigger, a new random element is chosen (which may be
% the same as the previous one)

%#codegen

persistent trigger_
persistent y_

if isempty(trigger_)
    trigger_=trigger; % This ensures that at the first timestep, an y is chosen
    getNewElement = 1;
    y_=0; % Will be overwritten a few lines later
else
    if trigger>trigger_
        getNewElement=1;
    else
        getNewElement=0;
    end;
    trigger_=trigger;
end;


if getNewElement
    y_ =u(randi(length(u)));
end;
y=y_;
